simulink model "analog_sensors_handler"  (R2021a)
settings: Solver=VariableStepAuto  StartTime=0.0  StopTime=10.0  RelTol=1e-3
libraries: simulink x1
settings Model: Creator=Intuito_PC  LastModifiedBy=Intuito_PC

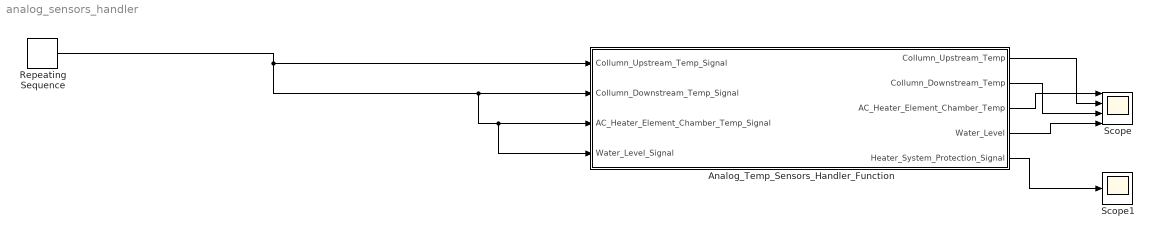
== system analog_sensors_handler ==
  Analog_Temp_Sensors_Handler_Function : MATLAB Function  TreatAsAtomicUnit=on
  Repeating Sequence : simulink/Sources/Repeating Sequence  rep_seq_t=[0 2]  rep_seq_y=[1 2013]
  Scope : Scope  NumInputPorts=4
  Scope1 : Scope
  wires:
  Analog_Temp_Sensors_Handler_Function/3(AC_Heater_Element_Chamber_Temp) -> Scope/1
  Analog_Temp_Sensors_Handler_Function/1(Collumn_Upstream_Temp) -> Scope/2
  Analog_Temp_Sensors_Handler_Function/2(Collumn_Downstream_Temp) -> Scope/3
  Analog_Temp_Sensors_Handler_Function/4(Water_Level) -> Scope/4
  Analog_Temp_Sensors_Handler_Function/5(Heater_System_Protection_Signal) -> Scope1/1
  Repeating Sequence/1 -> Analog_Temp_Sensors_Handler_Function/4(Water_Level_Signal), Analog_Temp_Sensors_Handler_Function/3(AC_Heater_Element_Chamber_Temp_Signal), Analog_Temp_Sensors_Handler_Function/2(Collumn_Downstream_Temp_Signal), Analog_Temp_Sensors_Handler_Function/1(Collumn_Upstream_Temp_Signal)

== matlab function analog_sensors_handler/Analog_Temp_Sensors_Handler_Function ==
  data: Collumn_Upstream_Temp_Signal input; Collumn_Upstream_Temp output; Collumn_Downstream_Temp_Signal input; AC_Heater_Element_Chamber_Temp_Signal input; Water_Level_Signal input; Collumn_Downstream_Temp output; AC_Heater_Element_Chamber_Temp output; Water_Level output; Heater_System_Protection_Signal output
function [Collumn_Upstream_Temp, Collumn_Downstream_Temp, AC_Heater_Element_Chamber_Temp, Water_Level, Heater_System_Protection_Signal] = fcn(Collumn_Upstream_Temp_Signal, Collumn_Downstream_Temp_Signal, AC_Heater_Element_Chamber_Temp_Signal, Water_Level_Signal)
% Analog Temp Sensors Constants
THERMISTORNOMINAL = 90000;
TEMPERATURENOMINAL = 298; % 25 dge_C
BCOEFFICIENT = 3950;
SERIESRESISTOR = 10000; % R_1

% Temp sensor 1
R_1 = SERIESRESISTOR*(Collumn_Upstream_Temp_Signal/1023)/(5 - (Collumn_Upstream_Temp_Signal/1023)*4.99); % NTC Resistance
Collumn_Upstream_Temp = 1/(1/TEMPERATURENOMINAL - log(abs(THERMISTORNOMINAL/R_1))/BCOEFFICIENT) -273; % Compute temp
% Temp sensor 2
R_2 = SERIESRESISTOR*(Collumn_Downstream_Temp_Signal/1023)/(5 - (Collumn_Downstream_Temp_Signal/1023)*4.99); % NTC Resistance
Collumn_Downstream_Temp = 1/(1/TEMPERATURENOMINAL - log(abs(THERMISTORNOMINAL/R_2))/BCOEFFICIENT) -273; % Compute temp
% Temp sensor 3
R_3 = SERIESRESISTOR*(AC_Heater_Element_Chamber_Temp_Signal/1023)/(5 - (AC_Heater_Element_Chamber_Temp_Signal/1023)*4.99); % NTC Resistance
AC_Heater_Element_Chamber_Temp = 1/(1/TEMPERATURENOMINAL - log(abs(THERMISTORNOMINAL/R_3))/BCOEFFICIENT) -273; % Compute temp

% Water level sensor
Water_Level = Water_Level_Signal/1023*100;

% Heater System Protection
if AC_Heater_Element_Chamber_Temp > 160
    Heater_System_Protection_Signal = 1;
else
    Heater_System_Protection_Signal = 0;
end
end
